simulink model "Nmpc_pathctl_casadi"  (R2022b)
settings: Solver=FixedStepAuto  StartTime=0.0  StopTime=433  FixedStep=.001  MaxStep=0.01  RelTol=1e-3
values from neighbouring files (symbols this model uses):
  xuanze = Input(15)    [NMPC_casadi_yhn.m]    (also in plotfig.m = 0)
libraries: Solver_SF x1
(part 2 of 11)

== matlab function Nmpc_pathctl_casadi/MATLAB Function1 ==
  data: V input; w input; z input; V0 output; lamada input; curvepos0 input; lateralPos0 input; theta0 input; w0 output; lamada0 output; z0 output; Flag output; target input
function [V0,w0, lamada0,z0,Flag]= fcn(V,w,z,lamada,curvepos0,lateralPos0,theta0,target)

V0 = V;
w0 = w;
lamada0 = lamada;
z0 = z;
%% 代入真实的车辆状态，为计算真实的轮胎侧偏角做准备
d = 1.55; %左右轮距
Lf = 1.05;%质心到前轴的距离
Lr = 1.61;%质心到后轴的距离
hcg = 0.54;%质心高度
Iz = 2059.2;%转动惯量
m = 1430;%质量
Iw = 16.8;%车轮转动惯量
Re = 0.3018;%轮胎自由半径
g = 9.8;%重力系数
K_air = 0.9;%空气阻力系数
A = 2.2;%迎风面积
rho_air = 1.206;%空气密度
K_roll = 0.002;%滚动阻力系数
c1f = 1.68;%前轮参数
c1r = 1.49;%后轮参数
c2f = 10.56;%前轮参数
c2r = 15.026;%后轮参数
c3f = 0.02;
c3r = 0.02;
Cy = 1;
Cy_dot = 0.1;
Cs_dot = 0.8;
Cz = 35;
Ctheta_dot = 1;
V_tar = 15;
h = 0.02;
eplim = 50;
epsilon=10^(-6);%epsilon is the tolerance;
min1=5; %min1 & max1 are minimum and maximum number of iterations;
max1=40;
Ep=0.05;%不知道这是什么，为了能跑起来，先设置为和老版一样
kk = 0;
%% 控制器参数
Delt_T =0.02; %[s]
N = 15; %% 15 cuts now delays a bit
Nc = 2;
%% 原有参考轨迹
shape=2.4;%参数名称，用于参考轨迹生成
dx1=25;dx2=21.95;%没有任何实际意义，只是参数名称
dy1=4.05;dy2=5.7;%没有任何实际意义，只是参数名称
Xs1=27.19;Xs2=56.46;%参数名称
N_point = 240;%点的个数
% control_points = [];
X_phi=1:1:N_point;%这个点的区间是根据纵向速度（x_dot）来定的，如果速度为10m/s则区间=10*0.1=1
z1=shape/dx1*(X_phi-Xs1)-shape/2;
z2=shape/dx2*(X_phi-Xs2)-shape/2;
Y_ref=dy1/2.*(1+tanh(z1))-dy2/2.*(1+tanh(z2));
gamma_s = atan2(Y_ref,X_phi);

%% 障碍物信息
    X_obstacle=zeros(1,1);
    X_obstacle(1)=30;

    Y_obstacle=zeros(1,1);
    Y_obstacle(1)=0.5;

%% 计算航向角导数
dot_gamma_s = zeros(N_point);
dot_dot_gamma_s = zeros(N_point);
for i=1:N_point-1
    dot_gamma_s(i) = gamma_s(i+1)-gamma_s(i);
end
    dot_gamma_s(N_point)=dot_gamma_s(N_point-1);
for i=1:N_point-1
    dot_dot_gamma_s(i) = dot_gamma_s(i+1)-dot_gamma_s(i);
end
    dot_dot_gamma_s(N_point)=dot_dot_gamma_s(N_point-1);
%% 寻找距离车辆最近的点
target_dist = sqrt((lateralPos0-Y_ref(target))^2 + (curvepos0-X_phi(target))^2);
for goal = target:target+10
    if goal>length(Y_ref)
        i = goal-length(Y_ref);
    else
        i =goal;
    end
    dist = sqrt((lateralPos0-Y_ref(target))^2 + (curvepos0-X_phi(target))^2);
    if dist < target_dist
        target = i;
        err = target_dist;
        target_dist = dist;
    end
    if dist < 0.07
        target = target+1;
        err = target_dist;
        break;
    end
end
%更新到曲线坐标系中
target0 = target;
curvepos0 = target;
lateralPos0 = target_dist;

%% 使用最优控制方法找到P1,P2,P3
x0 = [0,0,0];
V_dac = [x0(1),x0(2),x0(3);1,0,0;0,1,0;0,0,1];
[mm1,n] = size(V_dac);
Y = ones(n+1,1);
for mm = 1:n+1
    Z = V_dac(mm,1:n);
%==========================================================================下面展开函数myobj_f  ON    
x = Z;
P1 = x(1);
P2 = x(2);
P3 = x(3);
x1 = curvepos0;
x2 = lateralPos0;
x3 = theta0;

for j = 1:N
    fenmu = 1-x2*dot_gamma_s(floor(x1));
    fenzi_a = cos(x3-gamma_s(floor(x1)));
    fenzi_b = sin(x3-gamma_s(floor(x1)));
    %控制量更新
    %求解G(x0)
    H_V_a = 2*Cs_dot*(V0*fenzi_a/fenmu-V_tar)*fenzi_a/fenmu;
    H_V_b = 2*Cy_dot*(V0*fenzi_b^2);
    H_V_c = P1*fenzi_a/fenmu;
    H_V_d = P2*fenzi_b;
    H_V = H_V_a+H_V_b+H_V_c+H_V_d;
    H_w = 2*Ctheta_dot*w0+P3;
    H_z = -Cz/(z0+50)-2*lamada0*z0;
    H_lamada = (x1-30)^2/16+(x2-0.5)^2/4-1-z0^2;
    G_x0 = [H_V;H_w;H_z;H_lamada];
    %求解个G(x0+dotx)
    
    x1_tem = x1+Delt_T*V0*fenzi_a/fenmu;
    x2_tem = x2+Delt_T*V0*fenzi_b;
    x3_tem = x3+Delt_T*w0;
    fenmu_tem = 1-x2_tem*dot_gamma_s(floor(x1_tem));
    fenzi_a_tem = cos(x3_tem-gamma_s(floor(x1_tem)));
    fenzi_b_tem = sin(x3_tem-gamma_s(floor(x1_tem)));
    H_V_a = 2*Cs_dot*(V0*fenzi_a_tem/fenmu_tem-V_tar)*fenzi_a_tem/fenmu_tem;
    H_V_b = 2*Cy_dot*(V0*fenzi_b_tem^2);
    H_V_c = P1*fenzi_a_tem/fenmu_tem;
    H_V_d = P2*fenzi_b_tem;
    H_V_xdot = H_V_a+H_V_b+H_V_c+H_V_d;
    H_w_xdot = 2*Ctheta_dot*w0+P3;
    H_z_xdot = -Cz/(z0+eplim)-2*lamada0*z0;
    H_lamada_dot = (x1_tem-30)^2/16+(x2_tem-0.5)^2/4-1-z0^2;
    G_xdot = [H_V_xdot;H_w_xdot;H_z_xdot;H_lamada_dot];
    G_x_xdot = (G_xdot-G_x0)/0.02;
    %求解G对U的偏导
    G_U_a = 2*Cs_dot*(fenzi_a/fenmu)^2+2*Cy_dot*fenzi_b^2;
    G_U_b = 2*Ctheta_dot;
    G_U_c = -Cz/((z0+eplim)^2)-2*lamada0;
    G_U_d = -2*z0;
    G_U = [G_U_a,0,0,0;0,G_U_b,0,0;0,0,G_U_c,G_U_d;0,0,G_U_d,0];
    %求解u的导数
    dot_u = inv(G_U)*(-G_x_xdot-50*G_x0);
    V0 = V0+dot_u(1)*Delt_T;
    w0 = w0+dot_u(2)*Delt_T;
    z0 = z0+dot_u(3)*Delt_T;
    lamada0 = lamada0+dot_u(4)*Delt_T;
    %开始H对x1求偏导
    H_x1_a = 2*Cs_dot*(V0*fenzi_a/fenmu-V_tar)*(V0*fenzi_b/fenmu*dot_gamma_s(floor(x1))+V0*fenzi_a/fenmu^2*dot_dot_gamma_s(floor(x1)));
    H_x1_b = -2*Cy_dot*(V0^2*fenzi_b*fenzi_a*dot_gamma_s(floor(x1)));
    H_x1_c = P1*V0*fenzi_b/fenzi_a*dot_gamma_s(floor(x1))+V0*fenzi_a/fenmu^2*dot_dot_gamma_s(floor(x1));
    H_x1_d = -P2*V0*fenzi_a*dot_gamma_s(floor(x1));
    H_x1 = H_x1_b+H_x1_a+H_x1_c+H_x1_d;
    %开始H对x2求导
    H_x2_a = 2*Cs_dot*(V0*fenzi_a/fenmu-V_tar)*V0*fenzi_a/fenmu^2*dot_gamma_s(floor(x1));
    H_x2_b = 2*Cy*x2;
    H_x2_c = P1*V0*fenzi_a/fenmu*dot_gamma_s(floor(x1));
    H_x2_d = 2*lamada0*(x2-0.5)/4;
    H_x2 = H_x2_a+H_x2_b+H_x2_c+H_x2_d;
    %开始H对x3求导
    H_x3_a = -2*Cs_dot*(V0*fenzi_a/fenmu-V_tar)*fenzi_a/fenmu;
    H_x3_b = 2*Cy_dot*V0*fenzi_b^2;
    H_x3_c = P1*fenzi_a/fenmu;
    H_x3_d = P2*fenzi_b;
    H_x3 = H_x3_a+H_x3_b+H_x3_c+H_x3_d;
    %更新状态
    x1 = x1+Delt_T*V0*fenzi_a/fenmu;
    x2 = x2+Delt_T*V0*fenzi_b;
    x3 = x3+Delt_T*w0;
end
f = abs(P1)+abs(P2)+abs(P3);
%==========================================================================展开函数myobj_f  OFF
    Y(mm) = f;
end
[mm2,lo] = min(Y);
[mm,hi] = max(Y);
li = hi;
ho = lo;
for mm=1:n+1 %寻找次zuix点
    if mm~=lo && mm~=hi && Y(mm)<=Y(li)
        li=mm;
    end
    if mm~=hi && mm~=lo && Y(mm)>=Y(li)
        ho=mm;
    end
end
cnt=0;
%%开始Nelder-Mead algorithm
while (Y(hi)>Y(lo)+epsilon && cnt<max1) || cnt<min1
    S=zeros(1,n);
    for mm=1:n+1
        S=S+V_dac(mm,1:n);
    end
    M=(S-V_dac(hi,1:n))/n;
    R=2*M-V_dac(hi,1:n);
%==========================================================================下面展开函数myobj_f  ON
x=R;
P1 = x(1);
P2 = x(2);
P3 = x(3);
x1 = curvepos0;
x2 = lateralPos0;
x3 = theta0;
for j = 1:N
    fenmu = 1-x2*dot_gamma_s(floor(x1));
    fenzi_a = cos(x3-gamma_s(floor(x1)));
    fenzi_b = sin(x3-gamma_s(floor(x1)));
    %控制量更新
    %求解G(x0)
    H_V_a = 2*Cs_dot*(V0*fenzi_a/fenmu-V_tar)*fenzi_a/fenmu;
    H_V_b = 2*Cy_dot*(V0*fenzi_b^2);
    H_V_c = P1*fenzi_a/fenmu;
    H_V_d = P2*fenzi_b;
    H_V = H_V_a+H_V_b+H_V_c+H_V_d;
    H_w = 2*Ctheta_dot*w0+P3;
    H_z = -Cz/(z0+50)-2*lamada0*z0;
    H_lamada = (x1-30)^2/16+(x2-0.5)^2/4-1-z0^2;
    G_x0 = [H_V;H_w;H_z;H_lamada];
    %求解个G(x0+dotx)
    x1_tem = x1+Delt_T*V0*fenzi_a/fenmu;
    x2_tem = x2+Delt_T*V0*fenzi_b;
    x3_tem = x3+Delt_T*w0;
    fenmu_tem = 1-x2_tem*dot_gamma_s(floor(x1_tem));
    fenzi_a_tem = cos(x3_tem-gamma_s(floor(x1_tem)));
    fenzi_b_tem = sin(x3_tem-gamma_s(floor(x1_tem)));
    H_V_a = 2*Cs_dot*(V0*fenzi_a_tem/fenmu_tem-V_tar)*fenzi_a_tem/fenmu_tem;
    H_V_b = 2*Cy_dot*(V0*fenzi_b_tem^2);
    H_V_c = P1*fenzi_a_tem/fenmu_tem;
    H_V_d = P2*fenzi_b_tem;
    H_V_xdot = H_V_a+H_V_b+H_V_c+H_V_d;
    H_w_xdot = 2*Ctheta_dot*w0+P3;
    H_z_xdot = -Cz/(z0+eplim)-2*lamada0*z0;
    H_lamada_dot = (x1_tem-30)^2/16+(x2_tem-0.5)^2/4-1-z0^2;
    G_xdot = [H_V_xdot;H_w_xdot;H_z_xdot;H_lamada_dot];
    G_x_xdot = (G_xdot-G_x0)/0.02;
    %求解G对U的偏导
    G_U_a = 2*Cs_dot*(fenzi_a/fenmu)^2+2*Cy_dot*fenzi_b^2;
    G_U_b = 2*Ctheta_dot;
    G_U_c = -Cz/((z0+eplim)^2)-2*lamada0;
    G_U_d = -2*z0;
    G_U = [G_U_a,0,0,0;0,G_U_b,0,0;0,0,G_U_c,G_U_d;0,0,G_U_d,0];
    %求解u的导数
    dot_u = inv(G_U)*(-G_x_xdot-50*G_x0);
    V0 = V0+dot_u(1)*Delt_T;
    w0 = w0+dot_u(2)*Delt_T;
    z0 = z0+dot_u(3)*Delt_T;
    lamada0 = lamada0+dot_u(4)*Delt_T;
    %开始H对x1求偏导
    H_x1_a = 2*Cs_dot*(V0*fenzi_a/fenmu-V_tar)*(V0*fenzi_b/fenmu*dot_gamma_s(floor(x1))+V0*fenzi_a/fenmu^2*dot_dot_gamma_s(floor(x1)));
    H_x1_b = -2*Cy_dot*(V0^2*fenzi_b*fenzi_a*dot_gamma_s(floor(x1)));
    H_x1_c = P1*V0*fenzi_b/fenzi_a*dot_gamma_s(floor(x1))+V0*fenzi_a/fenmu^2*dot_dot_gamma_s(floor(x1));
    H_x1_d = -P2*V0*fenzi_a*dot_gamma_s(floor(x1));
    H_x1 = H_x1_b+H_x1_a+H_x1_c+H_x1_d;
    %开始H对x2求导
    H_x2_a = 2*Cs_dot*(V0*fenzi_a/fenmu-V_tar)*V0*fenzi_a/fenmu^2*dot_gamma_s(floor(x1));
    H_x2_b = 2*Cy*x2;
    H_x2_c = P1*V0*fenzi_a/fenmu*dot_gamma_s(floor(x1));
    H_x2_d = 2*lamada0*(x2-0.5)/4;
    H_x2 = H_x2_a+H_x2_b+H_x2_c+H_x2_d;
    %开始H对x3求导
    H_x3_a = -2*Cs_dot*(V0*fenzi_a/fenmu-V_tar)*fenzi_a/fenmu;
    H_x3_b = 2*Cy_dot*V0*fenzi_b^2;
    H_x3_c = P1*fenzi_a/fenmu;
    H_x3_d = P2*fenzi_b;
    H_x3 = H_x3_a+H_x3_b+H_x3_c+H_x3_d;
    %更新状态
    x1 = x1+Delt_T*V0*fenzi_a/fenmu;
    x2 = x2+Delt_T*V0*fenzi_b;
    x3 = x3+Delt_T*w0;
end
f = abs(P1)+abs(P2)+abs(P3);
%==========================================================================展开函数myobj_f  OFF
yR=f;
    if yR<Y(ho)
        if Y(li)<yR
            V_dac(hi,1:n)=R;
            Y(hi)=yR;
        else
            E=2*R-M;
%==========================================================================下面展开函数myobj_f  ON
x = E;
P1 = x(1);
P2 = x(2);
P3 = x(3);
x1 = curvepos0;
x2 = lateralPos0;
x3 = theta0;
for j = 1:N
    fenmu = 1-x2*dot_gamma_s(floor(x1));
    fenzi_a = cos(x3-gamma_s(floor(x1)));
    fenzi_b = sin(x3-gamma_s(floor(x1)));
    %控制量更新
    %求解G(x0)
    H_V_a = 2*Cs_dot*(V0*fenzi_a/fenmu-V_tar)*fenzi_a/fenmu;
    H_V_b = 2*Cy_dot*(V0*fenzi_b^2);
    H_V_c = P1*fenzi_a/fenmu;
    H_V_d = P2*fenzi_b;
    H_V = H_V_a+H_V_b+H_V_c+H_V_d;
    H_w = 2*Ctheta_dot*w0+P3;
    H_z = -Cz/(z0+50)-2*lamada0*z0;
    H_lamada = (x1-30)^2/16+(x2-0.5)^2/4-1-z0^2;
    G_x0 = [H_V;H_w;H_z;H_lamada];
    %求解个G(x0+dotx)
    x1_tem = x1+Delt_T*V0*fenzi_a/fenmu;
    x2_tem = x2+Delt_T*V0*fenzi_b;
    x3_tem = x3+Delt_T*w0;
    fenmu_tem = 1-x2_tem*dot_gamma_s(floor(x1_tem));
    fenzi_a_tem = cos(x3_tem-gamma_s(floor(x1_tem)));
    fenzi_b_tem = sin(x3_tem-gamma_s(floor(x1_tem)));
    H_V_a = 2*Cs_dot*(V0*fenzi_a_tem/fenmu_tem-V_tar)*fenzi_a_tem/fenmu_tem;
    H_V_b = 2*Cy_dot*(V0*fenzi_b_tem^2);
    H_V_c = P1*fenzi_a_tem/fenmu_tem;
    H_V_d = P2*fenzi_b_tem;
    H_V_xdot = H_V_a+H_V_b+H_V_c+H_V_d;
    H_w_xdot = 2*Ctheta_dot*w0+P3;
    H_z_xdot = -Cz/(z0+eplim)-2*lamada0*z0;
    H_lamada_dot = (x1_tem-30)^2/16+(x2_tem-0.5)^2/4-1-z0^2;
    G_xdot = [H_V_xdot;H_w_xdot;H_z_xdot;H_lamada_dot];
    G_x_xdot = (G_xdot-G_x0)/0.02;
    %求解G对U的偏导
    G_U_a = 2*Cs_dot*(fenzi_a/fenmu)^2+2*Cy_dot*fenzi_b^2;
    G_U_b = 2*Ctheta_dot;
    G_U_c = -Cz/((z0+eplim)^2)-2*lamada0;
    G_U_d = -2*z0;
    G_U = [G_U_a,0,0,0;0,G_U_b,0,0;0,0,G_U_c,G_U_d;0,0,G_U_d,0];
    %求解u的导数
    dot_u = inv(G_U)*(-G_x_xdot-50*G_x0);
    V0 = V0+dot_u(1)*Delt_T;
    w0 = w0+dot_u(2)*Delt_T;
    z0 = z0+dot_u(3)*Delt_T;
    lamada0 = lamada0+dot_u(4)*Delt_T;
    %开始H对x1求偏导
    H_x1_a = 2*Cs_dot*(V0*fenzi_a/fenmu-V_tar)*(V0*fenzi_b/fenmu*dot_gamma_s(floor(x1))+V0*fenzi_a/fenmu^2*dot_dot_gamma_s(floor(x1)));
    H_x1_b = -2*Cy_dot*(V0^2*fenzi_b*fenzi_a*dot_gamma_s(floor(x1)));
    H_x1_c = P1*V0*fenzi_b/fenzi_a*dot_gamma_s(floor(x1))+V0*fenzi_a/fenmu^2*dot_dot_gamma_s(floor(x1));
    H_x1_d = -P2*V0*fenzi_a*dot_gamma_s(floor(x1));
    H_x1 = H_x1_b+H_x1_a+H_x1_c+H_x1_d;
    %开始H对x2求导
    H_x2_a = 2*Cs_dot*(V0*fenzi_a/fenmu-V_tar)*V0*fenzi_a/fenmu^2*dot_gamma_s(floor(x1));
    H_x2_b = 2*Cy*x2;
    H_x2_c = P1*V0*fenzi_a/fenmu*dot_gamma_s(floor(x1));
    H_x2_d = 2*lamada0*(x2-0.5)/4;
    H_x2 = H_x2_a+H_x2_b+H_x2_c+H_x2_d;
    %开始H对x3求导
    H_x3_a = -2*Cs_dot*(V0*fenzi_a/fenmu-V_tar)*fenzi_a/fenmu;
    H_x3_b = 2*Cy_dot*V0*fenzi_b^2;
    H_x3_c = P1*fenzi_a/fenmu;
    H_x3_d = P2*fenzi_b;
    H_x3 = H_x3_a+H_x3_b+H_x3_c+H_x3_d;
    %更新状态
    x1 = x1+Delt_T*V0*fenzi_a/fenmu;
    x2 = x2+Delt_T*V0*fenzi_b;
    x3 = x3+Delt_T*w0;
end
f = abs(P1)+abs(P2)+abs(P3);
%==========================================================================展开函数myobj_f  OFF
            yE=f;
            if yE<Y(li)
                V_dac(hi,1:n)=E;
                Y(hi)=yE;
            else
                V_dac(hi,1:n)=R;
                Y(hi)=yR;
            end
        end
    else
        if yR<Y(hi)
            V_dac(hi,1:n)=R;
            Y(hi)=yR;
        end
        C1_dac=(V_dac(hi,1:n)+M)/2;
%==========================================================================下面展开函数myobj_f  ON
x=C1_dac;
P1 = x(1);
P2 = x(2);
P3 = x(3);
x1 = curvepos0;
x2 = lateralPos0;
x3 = theta0;
for j = 1:N
    fenmu = 1-x2*dot_gamma_s(floor(x1));
    fenzi_a = cos(x3-gamma_s(floor(x1)));
    fenzi_b = sin(x3-gamma_s(floor(x1)));
    %控制量更新
    %求解G(x0)
    H_V_a = 2*Cs_dot*(V0*fenzi_a/fenmu-V_tar)*fenzi_a/fenmu;
    H_V_b = 2*Cy_dot*(V0*fenzi_b^2);
    H_V_c = P1*fenzi_a/fenmu;
    H_V_d = P2*fenzi_b;
    H_V = H_V_a+H_V_b+H_V_c+H_V_d;
    H_w = 2*Ctheta_dot*w0+P3;
    H_z = -Cz/(z0+50)-2*lamada0*z0;
    H_lamada = (x1-30)^2/16+(x2-0.5)^2/4-1-z0^2;
    G_x0 = [H_V;H_w;H_z;H_lamada];
    %求解个G(x0+dotx)
    x1_tem = x1+Delt_T*V0*fenzi_a/fenmu;
    x2_tem = x2+Delt_T*V0*fenzi_b;
    x3_tem = x3+Delt_T*w0;
    fenmu_tem = 1-x2_tem*dot_gamma_s(floor(x1_tem));
    fenzi_a_tem = cos(x3_tem-gamma_s(floor(x1_tem)));
    fenzi_b_tem = sin(x3_tem-gamma_s(floor(x1_tem)));
    H_V_a = 2*Cs_dot*(V0*fenzi_a_tem/fenmu_tem-V_tar)*fenzi_a_tem/fenmu_tem;
    H_V_b = 2*Cy_dot*(V0*fenzi_b_tem^2);
    H_V_c = P1*fenzi_a_tem/fenmu_tem;
    H_V_d = P2*fenzi_b_tem;
    H_V_xdot = H_V_a+H_V_b+H_V_c+H_V_d;
    H_w_xdot = 2*Ctheta_dot*w0+P3;
    H_z_xdot = -Cz/(z0+eplim)-2*lamada0*z0;
    H_lamada_dot = (x1_tem-30)^2/16+(x2_tem-0.5)^2/4-1-z0^2;
    G_xdot = [H_V_xdot;H_w_xdot;H_z_xdot;H_lamada_dot];
    G_x_xdot = (G_xdot-G_x0)/0.02;
    %求解G对U的偏导
    G_U_a = 2*Cs_dot*(fenzi_a/fenmu)^2+2*Cy_dot*fenzi_b^2;
    G_U_b = 2*Ctheta_dot;
    G_U_c = -Cz/((z0+eplim)^2)-2*lamada0;
    G_U_d = -2*z0;
    G_U = [G_U_a,0,0,0;0,G_U_b,0,0;0,0,G_U_c,G_U_d;0,0,G_U_d,0];
    %求解u的导数
    dot_u = inv(G_U)*(-G_x_xdot-50*G_x0);
    V0 = V0+dot_u(1)*Delt_T;
    w0 = w0+dot_u(2)*Delt_T;
    z0 = z0+dot_u(3)*Delt_T;
    lamada0 = lamada0+dot_u(4)*Delt_T;
    %开始H对x1求偏导
    H_x1_a = 2*Cs_dot*(V0*fenzi_a/fenmu-V_tar)*(V0*fenzi_b/fenmu*dot_gamma_s(floor(x1))+V0*fenzi_a/fenmu^2*dot_dot_gamma_s(floor(x1)));
    H_x1_b = -2*Cy_dot*(V0^2*fenzi_b*fenzi_a*dot_gamma_s(floor(x1)));
    H_x1_c = P1*V0*fenzi_b/fenzi_a*dot_gamma_s(floor(x1))+V0*fenzi_a/fenmu^2*dot_dot_gamma_s(floor(x1));
    H_x1_d = -P2*V0*fenzi_a*dot_gamma_s(floor(x1));
    H_x1 = H_x1_b+H_x1_a+H_x1_c+H_x1_d;
    %开始H对x2求导
    H_x2_a = 2*Cs_dot*(V0*fenzi_a/fenmu-V_tar)*V0*fenzi_a/fenmu^2*dot_gamma_s(floor(x1));
    H_x2_b = 2*Cy*x2;
    H_x2_c = P1*V0*fenzi_a/fenmu*dot_gamma_s(floor(x1));
    H_x2_d = 2*lamada0*(x2-0.5)/4;
    H_x2 = H_x2_a+H_x2_b+H_x2_c+H_x2_d;
    %开始H对x3求导
    H_x3_a = -2*Cs_dot*(V0*fenzi_a/fenmu-V_tar)*fenzi_a/fenmu;
    H_x3_b = 2*Cy_dot*V0*fenzi_b^2;
    H_x3_c = P1*fenzi_a/fenmu;
    H_x3_d = P2*fenzi_b;
    H_x3 = H_x3_a+H_x3_b+H_x3_c+H_x3_d;
    %更新状态
    x1 = x1+Delt_T*V0*fenzi_a/fenmu;
    x2 = x2+Delt_T*V0*fenzi_b;
    x3 = x3+Delt_T*w0;
end
f = abs(P1)+abs(P2)+abs(P3);
%==========================================================================展开函数myobj_f  OFF
        yC1=f;
        C2_dac=(M+R)/2;
%==========================================================================下面展开函数myobj_f  ON
x=C2_dac;
P1 = x(1);
P2 = x(2);
P3 = x(3);
x1 = curvepos0;
x2 = lateralPos0;
x3 = theta0;
for j = 1:N
    fenmu = 1-x2*dot_gamma_s(floor(x1));
    fenzi_a = cos(x3-gamma_s(floor(x1)));
    fenzi_b = sin(x3-gamma_s(floor(x1)));
    %控制量更新
    %求解G(x0)
    H_V_a = 2*Cs_dot*(V0*fenzi_a/fenmu-V_tar)*fenzi_a/fenmu;
    H_V_b = 2*Cy_dot*(V0*fenzi_b^2);
    H_V_c = P1*fenzi_a/fenmu;
    H_V_d = P2*fenzi_b;
    H_V = H_V_a+H_V_b+H_V_c+H_V_d;
    H_w = 2*Ctheta_dot*w0+P3;
    H_z = -Cz/(z0+50)-2*lamada0*z0;
    H_lamada = (x1-30)^2/16+(x2-0.5)^2/4-1-z0^2;
    G_x0 = [H_V;H_w;H_z;H_lamada];
    %求解个G(x0+dotx)
    x1_tem = x1+Delt_T*V0*fenzi_a/fenmu;
    x2_tem = x2+Delt_T*V0*fenzi_b;
    x3_tem = x3+Delt_T*w0;
    fenmu_tem = 1-x2_tem*dot_gamma_s(floor(x1_tem));
    fenzi_a_tem = cos(x3_tem-gamma_s(floor(x1_tem)));
    fenzi_b_tem = sin(x3_tem-gamma_s(floor(x1_tem)));
    H_V_a = 2*Cs_dot*(V0*fenzi_a_tem/fenmu_tem-V_tar)*fenzi_a_tem/fenmu_tem;
    H_V_b = 2*Cy_dot*(V0*fenzi_b_tem^2);
    H_V_c = P1*fenzi_a_tem/fenmu_tem;
    H_V_d = P2*fenzi_b_tem;
    H_V_xdot = H_V_a+H_V_b+H_V_c+H_V_d;
    H_w_xdot = 2*Ctheta_dot*w0+P3;
    H_z_xdot = -Cz/(z0+eplim)-2*lamada0*z0;
    H_lamada_dot = (x1_tem-30)^2/16+(x2_tem-0.5)^2/4-1-z0^2;
    G_xdot = [H_V_xdot;H_w_xdot;H_z_xdot;H_lamada_dot];
    G_x_xdot = (G_xdot-G_x0)/0.02;
    %求解G对U的偏导
    G_U_a = 2*Cs_dot*(fenzi_a/fenmu)^2+2*Cy_dot*fenzi_b^2;
    G_U_b = 2*Ctheta_dot;
    G_U_c = -Cz/((z0+eplim)^2)-2*lamada0;
    G_U_d = -2*z0;
    G_U = [G_U_a,0,0,0;0,G_U_b,0,0;0,0,G_U_c,G_U_d;0,0,G_U_d,0];
    %求解u的导数
    dot_u = inv(G_U)*(-G_x_xdot-50*G_x0);
    V0 = V0+dot_u(1)*Delt_T;
    w0 = w0+dot_u(2)*Delt_T;
    z0 = z0+dot_u(3)*Delt_T;
    lamada0 = lamada0+dot_u(4)*Delt_T;
    %开始H对x1求偏导
    H_x1_a = 2*Cs_dot*(V0*fenzi_a/fenmu-V_tar)*(V0*fenzi_b/fenmu*dot_gamma_s(floor(x1))+V0*fenzi_a/fenmu^2*dot_dot_gamma_s(floor(x1)));
    H_x1_b = -2*Cy_dot*(V0^2*fenzi_b*fenzi_a*dot_gamma_s(floor(x1)));
    H_x1_c = P1*V0*fenzi_b/fenzi_a*dot_gamma_s(floor(x1))+V0*fenzi_a/fenmu^2*dot_dot_gamma_s(floor(x1));
    H_x1_d = -P2*V0*fenzi_a*dot_gamma_s(floor(x1));
    H_x1 = H_x1_b+H_x1_a+H_x1_c+H_x1_d;
    %开始H对x2求导
    H_x2_a = 2*Cs_dot*(V0*fenzi_a/fenmu-V_tar)*V0*fenzi_a/fenmu^2*dot_gamma_s(floor(x1));
    H_x2_b = 2*Cy*x2;
    H_x2_c = P1*V0*fenzi_a/fenmu*dot_gamma_s(floor(x1));
    H_x2_d = 2*lamada0*(x2-0.5)/4;
    H_x2 = H_x2_a+H_x2_b+H_x2_c+H_x2_d;
    %开始H对x3求导
    H_x3_a = -2*Cs_dot*(V0*fenzi_a/fenmu-V_tar)*fenzi_a/fenmu;
    H_x3_b = 2*Cy_dot*V0*fenzi_b^2;
    H_x3_c = P1*fenzi_a/fenmu;
    H_x3_d = P2*fenzi_b;
    H_x3 = H_x3_a+H_x3_b+H_x3_c+H_x3_d;
    %更新状态
    x1 = x1+Delt_T*V0*fenzi_a/fenmu;
    x2 = x2+Delt_T*V0*fenzi_b;
    x3 = x3+Delt_T*w0;
end
f = abs(P1)+abs(P2)+abs(P3);
%==========================================================================展开函数myobj_f  OFF
        yC2=f;
        if yC2<yC1
            C1_dac=C2_dac;
            yC1=yC2;
        end
        if yC1<Y(hi)
            V_dac(hi,1:n)=C1_dac;
            Y(hi)=yC1;
        else
            for mm=1:n+1
                if mm~=lo
                    V_dac(mm,1:n)=(V_dac(mm,1:n)+V_dac(lo,1:n))/2;
                    Z=V_dac(mm,1:n);
%==========================================================================下面展开函数myobj_f  ON
x=Z;
P1 = x(1);
P2 = x(2);
P3 = x(3);
x1 = curvepos0;
x2 = lateralPos0;
x3 = theta0;
for j = 1:N
    fenmu = 1-x2*dot_gamma_s(floor(x1));
    fenzi_a = cos(x3-gamma_s(floor(x1)));
    fenzi_b = sin(x3-gamma_s(floor(x1)));
    %控制量更新
    %求解G(x0)
    H_V_a = 2*Cs_dot*(V0*fenzi_a/fenmu-V_tar)*fenzi_a/fenmu;
    H_V_b = 2*Cy_dot*(V0*fenzi_b^2);
    H_V_c = P1*fenzi_a/fenmu;
    H_V_d = P2*fenzi_b;
    H_V = H_V_a+H_V_b+H_V_c+H_V_d;
    H_w = 2*Ctheta_dot*w0+P3;
    H_z = -Cz/(z0+50)-2*lamada0*z0;
    H_lamada = (x1-30)^2/16+(x2-0.5)^2/4-1-z0^2;
    G_x0 = [H_V;H_w;H_z;H_lamada];
    %求解个G(x0+dotx)
    x1_tem = x1+Delt_T*V0*fenzi_a/fenmu;
    x2_tem = x2+Delt_T*V0*fenzi_b;
    x3_tem = x3+Delt_T*w0;
    fenmu_tem = 1-x2_tem*dot_gamma_s(floor(x1_tem));
    fenzi_a_tem = cos(x3_tem-gamma_s(floor(x1_tem)));
    fenzi_b_tem = sin(x3_tem-gamma_s(floor(x1_tem)));
    H_V_a = 2*Cs_dot*(V0*fenzi_a_tem/fenmu_tem-V_tar)*fenzi_a_tem/fenmu_tem;
    H_V_b = 2*Cy_dot*(V0*fenzi_b_tem^2);
    H_V_c = P1*fenzi_a_tem/fenmu_tem;
    H_V_d = P2*fenzi_b_tem;
    H_V_xdot = H_V_a+H_V_b+H_V_c+H_V_d;
    H_w_xdot = 2*Ctheta_dot*w0+P3;
    H_z_xdot = -Cz/(z0+eplim)-2*lamada0*z0;
    H_lamada_dot = (x1_tem-30)^2/16+(x2_tem-0.5)^2/4-1-z0^2;
    G_xdot = [H_V_xdot;H_w_xdot;H_z_xdot;H_lamada_dot];
    G_x_xdot = (G_xdot-G_x0)/0.02;
    %求解G对U的偏导
    G_U_a = 2*Cs_dot*(fenzi_a/fenmu)^2+2*Cy_dot*fenzi_b^2;
    G_U_b = 2*Ctheta_dot;
    G_U_c = -Cz/((z0+eplim)^2)-2*lamada0;
    G_U_d = -2*z0;
    G_U = [G_U_a,0,0,0;0,G_U_b,0,0;0,0,G_U_c,G_U_d;0,0,G_U_d,0];
    %求解u的导数
    dot_u = inv(G_U)*(-G_x_xdot-50*G_x0);
    V0 = V0+dot_u(1)*Delt_T;
    w0 = w0+dot_u(2)*Delt_T;
    z0 = z0+dot_u(3)*Delt_T;
    lamada0 = lamada0+dot_u(4)*Delt_T;
    %开始H对x1求偏导
    H_x1_a = 2*Cs_dot*(V0*fenzi_a/fenmu-V_tar)*(V0*fenzi_b/fenmu*dot_gamma_s(floor(x1))+V0*fenzi_a/fenmu^2*dot_dot_gamma_s(floor(x1)));
    H_x1_b = -2*Cy_dot*(V0^2*fenzi_b*fenzi_a*dot_gamma_s(floor(x1)));
    H_x1_c = P1*V0*fenzi_b/fenzi_a*dot_gamma_s(floor(x1))+V0*fenzi_a/fenmu^2*dot_dot_gamma_s(floor(x1));
    H_x1_d = -P2*V0*fenzi_a*dot_gamma_s(floor(x1));
    H_x1 = H_x1_b+H_x1_a+H_x1_c+H_x1_d;
    %开始H对x2求导
    H_x2_a = 2*Cs_dot*(V0*fenzi_a/fenmu-V_tar)*V0*fenzi_a/fenmu^2*dot_gamma_s(floor(x1));
    H_x2_b = 2*Cy*x2;
    H_x2_c = P1*V0*fenzi_a/fenmu*dot_gamma_s(floor(x1));
    H_x2_d = 2*lamada0*(x2-0.5)/4;
    H_x2 = H_x2_a+H_x2_b+H_x2_c+H_x2_d;
    %开始H对x3求导
    H_x3_a = -2*Cs_dot*(V0*fenzi_a/fenmu-V_tar)*fenzi_a/fenmu;
    H_x3_b = 2*Cy_dot*V0*fenzi_b^2;
    H_x3_c = P1*fenzi_a/fenmu;
    H_x3_d = P2*fenzi_b;
    H_x3 = H_x3_a+H_x3_b+H_x3_c+H_x3_d;
    %更新状态
    x1 = x1+Delt_T*V0*fenzi_a/fenmu;
    x2 = x2+Delt_T*V0*fenzi_b;
    x3 = x3+Delt_T*w0;
end
f = abs(P1)+abs(P2)+abs(P3);
%==========================================================================展开函数myobj_f  OFF
                    Y(mm)=f;
                end
            end
        end
    end
    [mm4,lo]=min(Y);
    [mm5,hi]=max(Y);
    li=hi;
    ho=lo;
    for mm=1:n+1
        if mm~=lo && mm~=hi && Y(mm)<=Y(li)
            li=mm;
        end
        if mm~=hi && mm~=lo && Y(mm)>=Y(li)
            ho=mm;
        end
    end
    cnt=cnt+1;   
end
snorm=0;   
for mm=1:n
    s=norm(V_dac(mm)-V_dac(lo));
    if s>=snorm
        snorm=s; 
    end
end
Re=[V_dac(lo,1:n) cnt];
%==========================================================================下面展开函数myobj_f  ON  
x=[Re(1),Re(2),Re(3)];
P1 = x(1);
P2 = x(2);
P3 = x(3);
x1 = curvepos0;
x2 = lateralPos0;
x3 = theta0;
for j = 1:N
    fenmu = 1-x2*dot_gamma_s(floor(x1));
    fenzi_a = cos(x3-gamma_s(floor(x1)));
    fenzi_b = sin(x3-gamma_s(floor(x1)));
    %控制量更新
    %求解G(x0)
    H_V_a = 2*Cs_dot*(V0*fenzi_a/fenmu-V_tar)*fenzi_a/fenmu;
    H_V_b = 2*Cy_dot*(V0*fenzi_b^2);
    H_V_c = P1*fenzi_a/fenmu;
    H_V_d = P2*fenzi_b;
    H_V = H_V_a+H_V_b+H_V_c+H_V_d;
    H_w = 2*Ctheta_dot*w0+P3;
    H_z = -Cz/(z0+50)-2*lamada0*z0;
    H_lamada = (x1-30)^2/16+(x2-0.5)^2/4-1-z0^2;
    G_x0 = [H_V;H_w;H_z;H_lamada];
    %求解个G(x0+dotx)
    x1_tem = x1+Delt_T*V0*fenzi_a/fenmu;
    x2_tem = x2+Delt_T*V0*fenzi_b;
    x3_tem = x3+Delt_T*w0;
    fenmu_tem = 1-x2_tem*dot_gamma_s(floor(x1_tem));
    fenzi_a_tem = cos(x3_tem-gamma_s(floor(x1_tem)));
    fenzi_b_tem = sin(x3_tem-gamma_s(floor(x1_tem)));
    H_V_a = 2*Cs_dot*(V0*fenzi_a_tem/fenmu_tem-V_tar)*fenzi_a_tem/fenmu_tem;
    H_V_b = 2*Cy_dot*(V0*fenzi_b_tem^2);
    H_V_c = P1*fenzi_a_tem/fenmu_tem;
    H_V_d = P2*fenzi_b_tem;
    H_V_xdot = H_V_a+H_V_b+H_V_c+H_V_d;
    H_w_xdot = 2*Ctheta_dot*w0+P3;
    H_z_xdot = -Cz/(z0+eplim)-2*lamada0*z0;
    H_lamada_dot = (x1_tem-30)^2/16+(x2_tem-0.5)^2/4-1-z0^2;
    G_xdot = [H_V_xdot;H_w_xdot;H_z_xdot;H_lamada_dot];
    G_x_xdot = (G_xdot-G_x0)/0.02;
    %求解G对U的偏导
    G_U_a = 2*Cs_dot*(fenzi_a/fenmu)^2+2*Cy_dot*fenzi_b^2;
    G_U_b = 2*Ctheta_dot;
    G_U_c = -Cz/((z0+eplim)^2)-2*lamada0;
    G_U_d = -2*z0;
    G_U = [G_U_a,0,0,0;0,G_U_b,0,0;0,0,G_U_c,G_U_d;0,0,G_U_d,0];
    %求解u的导数
    dot_u = inv(G_U)*(-G_x_xdot-50*G_x0);
    V0 = V0+dot_u(1)*Delt_T;
    w0 = w0+dot_u(2)*Delt_T;
    z0 = z0+dot_u(3)*Delt_T;
    lamada0 = lamada0+dot_u(4)*Delt_T;
    %开始H对x1求偏导
    H_x1_a = 2*Cs_dot*(V0*fenzi_a/fenmu-V_tar)*(V0*fenzi_b/fenmu*dot_gamma_s(floor(x1))+V0*fenzi_a/fenmu^2*dot_dot_gamma_s(floor(x1)));
    H_x1_b = -2*Cy_dot*(V0^2*fenzi_b*fenzi_a*dot_gamma_s(floor(x1)));
    H_x1_c = P1*V0*fenzi_b/fenzi_a*dot_gamma_s(floor(x1))+V0*fenzi_a/fenmu^2*dot_dot_gamma_s(floor(x1));
    H_x1_d = -P2*V0*fenzi_a*dot_gamma_s(floor(x1));
    H_x1 = H_x1_b+H_x1_a+H_x1_c+H_x1_d;
    %开始H对x2求导
    H_x2_a = 2*Cs_dot*(V0*fenzi_a/fenmu-V_tar)*V0*fenzi_a/fenmu^2*dot_gamma_s(floor(x1));
    H_x2_b = 2*Cy*x2;
    H_x2_c = P1*V0*fenzi_a/fenmu*dot_gamma_s(floor(x1));
    H_x2_d = 2*lamada0*(x2-0.5)/4;
    H_x2 = H_x2_a+H_x2_b+H_x2_c+H_x2_d;
    %开始H对x3求导
    H_x3_a = -2*Cs_dot*(V0*fenzi_a/fenmu-V_tar)*fenzi_a/fenmu;
    H_x3_b = 2*Cy_dot*V0*fenzi_b^2;
    H_x3_c = P1*fenzi_a/fenmu;
    H_x3_d = P2*fenzi_b;
    H_x3 = H_x3_a+H_x3_b+H_x3_c+H_x3_d;
    %更新状态
    x1 = x1+Delt_T*V0*fenzi_a/fenmu;
    x2 = x2+Delt_T*V0*fenzi_b;
    x3 = x3+Delt_T*w0;
end
f = abs(P1)+abs(P2)+abs(P3);
a1 = f;
x_opt1=[Re(1),Re(2),Re(3)];
%==========================================================================展开函数myobj_f  OFF
%% 上面为一个计算循环
if(a1<=Ep)
    x_opt=x_opt1;
    Result_OB=a1;
else %第二个计算循环
    x0=[-1,1,-1];
    V_dac=[x0(1),x0(2),x0(3);1,0,0;0,1,0;0,0,1]; %V_dac is a 3 x n matrix containing starting simplex;
    [mm1 n]=size(V_dac);
% Order the V_dacertices
    Y=ones(n+1,1);
    for mm=1:n+1
        Z=V_dac(mm,1:n);
%==========================================================================下面展开函数myobj_f  ON
x=Z;
P1 = x(1);
P2 = x(2);
P3 = x(3);
x1 = curvepos0;
x2 = lateralPos0;
x3 = theta0;
for j = 1:N
    fenmu = 1-x2*dot_gamma_s(floor(x1));
    fenzi_a = cos(x3-gamma_s(floor(x1)));
    fenzi_b = sin(x3-gamma_s(floor(x1)));
    %控制量更新
    %求解G(x0)
    H_V_a = 2*Cs_dot*(V0*fenzi_a/fenmu-V_tar)*fenzi_a/fenmu;
    H_V_b = 2*Cy_dot*(V0*fenzi_b^2);
    H_V_c = P1*fenzi_a/fenmu;
    H_V_d = P2*fenzi_b;
    H_V = H_V_a+H_V_b+H_V_c+H_V_d;
    H_w = 2*Ctheta_dot*w0+P3;
    H_z = -Cz/(z0+50)-2*lamada0*z0;
    H_lamada = (x1-30)^2/16+(x2-0.5)^2/4-1-z0^2;
    G_x0 = [H_V;H_w;H_z;H_lamada];
    %求解个G(x0+dotx)
    x1_tem = x1+Delt_T*V0*fenzi_a/fenmu;
    x2_tem = x2+Delt_T*V0*fenzi_b;
    x3_tem = x3+Delt_T*w0;
    fenmu_tem = 1-x2_tem*dot_gamma_s(floor(x1_tem));
    fenzi_a_tem = cos(x3_tem-gamma_s(floor(x1_tem)));
    fenzi_b_tem = sin(x3_tem-gamma_s(floor(x1_tem)));
    H_V_a = 2*Cs_dot*(V0*fenzi_a_tem/fenmu_tem-V_tar)*fenzi_a_tem/fenmu_tem;
    H_V_b = 2*Cy_dot*(V0*fenzi_b_tem^2);
    H_V_c = P1*fenzi_a_tem/fenmu_tem;
    H_V_d = P2*fenzi_b_tem;
    H_V_xdot = H_V_a+H_V_b+H_V_c+H_V_d;
    H_w_xdot = 2*Ctheta_dot*w0+P3;
    H_z_xdot = -Cz/(z0+eplim)-2*lamada0*z0;
    H_lamada_dot = (x1_tem-30)^2/16+(x2_tem-0.5)^2/4-1-z0^2;
    G_xdot = [H_V_xdot;H_w_xdot;H_z_xdot;H_lamada_dot];
    G_x_xdot = (G_xdot-G_x0)/0.02;
    %求解G对U的偏导
    G_U_a = 2*Cs_dot*(fenzi_a/fenmu)^2+2*Cy_dot*fenzi_b^2;
    G_U_b = 2*Ctheta_dot;
    G_U_c = -Cz/((z0+eplim)^2)-2*lamada0;
    G_U_d = -2*z0;
    G_U = [G_U_a,0,0,0;0,G_U_b,0,0;0,0,G_U_c,G_U_d;0,0,G_U_d,0];
    %求解u的导数
    dot_u = inv(G_U)*(-G_x_xdot-50*G_x0);
    V0 = V0+dot_u(1)*Delt_T;
    w0 = w0+dot_u(2)*Delt_T;
    z0 = z0+dot_u(3)*Delt_T;
    lamada0 = lamada0+dot_u(4)*Delt_T;
    %开始H对x1求偏导
    H_x1_a = 2*Cs_dot*(V0*fenzi_a/fenmu-V_tar)*(V0*fenzi_b/fenmu*dot_gamma_s(floor(x1))+V0*fenzi_a/fenmu^2*dot_dot_gamma_s(floor(x1)));
    H_x1_b = -2*Cy_dot*(V0^2*fenzi_b*fenzi_a*dot_gamma_s(floor(x1)));
    H_x1_c = P1*V0*fenzi_b/fenzi_a*dot_gamma_s(floor(x1))+V0*fenzi_a/fenmu^2*dot_dot_gamma_s(floor(x1));
    H_x1_d = -P2*V0*fenzi_a*dot_gamma_s(floor(x1));
    H_x1 = H_x1_b+H_x1_a+H_x1_c+H_x1_d;
    %开始H对x2求导
    H_x2_a = 2*Cs_dot*(V0*fenzi_a/fenmu-V_tar)*V0*fenzi_a/fenmu^2*dot_gamma_s(floor(x1));
    H_x2_b = 2*Cy*x2;
    H_x2_c = P1*V0*fenzi_a/fenmu*dot_gamma_s(floor(x1));
    H_x2_d = 2*lamada0*(x2-0.5)/4;
    H_x2 = H_x2_a+H_x2_b+H_x2_c+H_x2_d;
    %开始H对x3求导
    H_x3_a = -2*Cs_dot*(V0*fenzi_a/fenmu-V_tar)*fenzi_a/fenmu;
    H_x3_b = 2*Cy_dot*V0*fenzi_b^2;
    H_x3_c = P1*fenzi_a/fenmu;
    H_x3_d = P2*fenzi_b;
    H_x3 = H_x3_a+H_x3_b+H_x3_c+H_x3_d;
    %更新状态
    x1 = x1+Delt_T*V0*fenzi_a/fenmu;
    x2 = x2+Delt_T*V0*fenzi_b;
    x3 = x3+Delt_T*w0;
end
f = abs(P1)+abs(P2)+abs(P3);
%==========================================================================展开函数myobj_f  OFF
        Y(mm)=f;
    end
    [mm2 lo]=min(Y);
    [mm3 hi]=max(Y);
    li=hi;
    ho=lo;
    for mm=1:n+1
        if mm~=lo && mm~=hi && Y(mm)<=Y(li)
            li=mm;
        end
        if mm~=hi && mm~=lo && Y(mm)>=Y(li)
            ho=mm;
        end
    end
    cnt=0;
%Start of Nelder-Mead algorithm
    while (Y(hi)>Y(lo)+epsilon && cnt<max1) || cnt<min1
        S=zeros(1,n);
        for mm=1:n+1
            S=S+V_dac(mm,1:n);
        end
        M=(S-V_dac(hi,1:n))/n;
        R=2*M-V_dac(hi,1:n);
%==========================================================================下面展开函数myobj_f  ON
x=R;
P1 = x(1);
P2 = x(2);
P3 = x(3);
x1 = curvepos0;
x2 = lateralPos0;
x3 = theta0;
for j = 1:N
    fenmu = 1-x2*dot_gamma_s(floor(x1));
    fenzi_a = cos(x3-gamma_s(floor(x1)));
    fenzi_b = sin(x3-gamma_s(floor(x1)));
    %控制量更新
    %求解G(x0)
    H_V_a = 2*Cs_dot*(V0*fenzi_a/fenmu-V_tar)*fenzi_a/fenmu;
    H_V_b = 2*Cy_dot*(V0*fenzi_b^2);
    H_V_c = P1*fenzi_a/fenmu;
    H_V_d = P2*fenzi_b;
    H_V = H_V_a+H_V_b+H_V_c+H_V_d;
    H_w = 2*Ctheta_dot*w0+P3;
    H_z = -Cz/(z0+50)-2*lamada0*z0;
    H_lamada = (x1-30)^2/16+(x2-0.5)^2/4-1-z0^2;
    G_x0 = [H_V;H_w;H_z;H_lamada];
    %求解个G(x0+dotx)
    x1_tem = x1+Delt_T*V0*fenzi_a/fenmu;
    x2_tem = x2+Delt_T*V0*fenzi_b;
    x3_tem = x3+Delt_T*w0;
    fenmu_tem = 1-x2_tem*dot_gamma_s(floor(x1_tem));
    fenzi_a_tem = cos(x3_tem-gamma_s(floor(x1_tem)));
    fenzi_b_tem = sin(x3_tem-gamma_s(floor(x1_tem)));
    H_V_a = 2*Cs_dot*(V0*fenzi_a_tem/fenmu_tem-V_tar)*fenzi_a_tem/fenmu_tem;
    H_V_b = 2*Cy_dot*(V0*fenzi_b_tem^2);
    H_V_c = P1*fenzi_a_tem/fenmu_tem;
    H_V_d = P2*fenzi_b_tem;
    H_V_xdot = H_V_a+H_V_b+H_V_c+H_V_d;
    H_w_xdot = 2*Ctheta_dot*w0+P3;
    H_z_xdot = -Cz/(z0+eplim)-2*lamada0*z0;
    H_lamada_dot = (x1_tem-30)^2/16+(x2_tem-0.5)^2/4-1-z0^2;
    G_xdot = [H_V_xdot;H_w_xdot;H_z_xdot;H_lamada_dot];
    G_x_xdot = (G_xdot-G_x0)/0.02;
    %求解G对U的偏导
    G_U_a = 2*Cs_dot*(fenzi_a/fenmu)^2+2*Cy_dot*fenzi_b^2;
    G_U_b = 2*Ctheta_dot;
    G_U_c = -Cz/((z0+eplim)^2)-2*lamada0;
    G_U_d = -2*z0;
    G_U = [G_U_a,0,0,0;0,G_U_b,0,0;0,0,G_U_c,G_U_d;0,0,G_U_d,0];
    %求解u的导数
    dot_u = inv(G_U)*(-G_x_xdot-50*G_x0);
    V0 = V0+dot_u(1)*Delt_T;
    w0 = w0+dot_u(2)*Delt_T;
    z0 = z0+dot_u(3)*Delt_T;
    lamada0 = lamada0+dot_u(4)*Delt_T;
    %开始H对x1求偏导
    H_x1_a = 2*Cs_dot*(V0*fenzi_a/fenmu-V_tar)*(V0*fenzi_b/fenmu*dot_gamma_s(floor(x1))+V0*fenzi_a/fenmu^2*dot_dot_gamma_s(floor(x1)));
    H_x1_b = -2*Cy_dot*(V0^2*fenzi_b*fenzi_a*dot_gamma_s(floor(x1)));
    H_x1_c = P1*V0*fenzi_b/fenzi_a*dot_gamma_s(floor(x1))+V0*fenzi_a/fenmu^2*dot_dot_gamma_s(floor(x1));
    H_x1_d = -P2*V0*fenzi_a*dot_gamma_s(floor(x1));
    H_x1 = H_x1_b+H_x1_a+H_x1_c+H_x1_d;
    %开始H对x2求导
    H_x2_a = 2*Cs_dot*(V0*fenzi_a/fenmu-V_tar)*V0*fenzi_a/fenmu^2*dot_gamma_s(floor(x1));
    H_x2_b = 2*Cy*x2;
    H_x2_c = P1*V0*fenzi_a/fenmu*dot_gamma_s(floor(x1));
    H_x2_d = 2*lamada0*(x2-0.5)/4;
    H_x2 = H_x2_a+H_x2_b+H_x2_c+H_x2_d;
    %开始H对x3求导
    H_x3_a = -2*Cs_dot*(V0*fenzi_a/fenmu-V_tar)*fenzi_a/fenmu;
    H_x3_b = 2*Cy_dot*V0*fenzi_b^2;
    H_x3_c = P1*fenzi_a/fenmu;
    H_x3_d = P2*fenzi_b;
    H_x3 = H_x3_a+H_x3_b+H_x3_c+H_x3_d;
    %更新状态
    x1 = x1+Delt_T*V0*fenzi_a/fenmu;
    x2 = x2+Delt_T*V0*fenzi_b;
    x3 = x3+Delt_T*w0;
end
f = abs(P1)+abs(P2)+abs(P3);
%==========================================================================展开函数myobj_f  OFF
        yR=f;
        if yR<Y(ho)
            if Y(li)<yR
                V_dac(hi,1:n)=R;
                Y(hi)=yR;
            else
                E=2*R-M;
%==========================================================================下面展开函数myobj_f  ON
x=E;
P1 = x(1);
P2 = x(2);
P3 = x(3);
x1 = curvepos0;
x2 = lateralPos0;
x3 = theta0;
for j = 1:N
    fenmu = 1-x2*dot_gamma_s(floor(x1));
    fenzi_a = cos(x3-gamma_s(floor(x1)));
    fenzi_b = sin(x3-gamma_s(floor(x1)));
    %控制量更新
    %求解G(x0)
    H_V_a = 2*Cs_dot*(V0*fenzi_a/fenmu-V_tar)*fenzi_a/fenmu;
    H_V_b = 2*Cy_dot*(V0*fenzi_b^2);
    H_V_c = P1*fenzi_a/fenmu;
    H_V_d = P2*fenzi_b;
    H_V = H_V_a+H_V_b+H_V_c+H_V_d;
    H_w = 2*Ctheta_dot*w0+P3;
    H_z = -Cz/(z0+50)-2*lamada0*z0;
    H_lamada = (x1-30)^2/16+(x2-0.5)^2/4-1-z0^2;
    G_x0 = [H_V;H_w;H_z;H_lamada];
    %求解个G(x0+dotx)
    x1_tem = x1+Delt_T*V0*fenzi_a/fenmu;
    x2_tem = x2+Delt_T*V0*fenzi_b;
    x3_tem = x3+Delt_T*w0;
    fenmu_tem = 1-x2_tem*dot_gamma_s(floor(x1_tem));
    fenzi_a_tem = cos(x3_tem-gamma_s(floor(x1_tem)));
    fenzi_b_tem = sin(x3_tem-gamma_s(floor(x1_tem)));
    H_V_a = 2*Cs_dot*(V0*fenzi_a_tem/fenmu_tem-V_tar)*fenzi_a_tem/fenmu_tem;
    H_V_b = 2*Cy_dot*(V0*fenzi_b_tem^2);
    H_V_c = P1*fenzi_a_tem/fenmu_tem;
    H_V_d = P2*fenzi_b_tem;
    H_V_xdot = H_V_a+H_V_b+H_V_c+H_V_d;
    H_w_xdot = 2*Ctheta_dot*w0+P3;
    H_z_xdot = -Cz/(z0+eplim)-2*lamada0*z0;
    H_lamada_dot = (x1_tem-30)^2/16+(x2_tem-0.5)^2/4-1-z0^2;
    G_xdot = [H_V_xdot;H_w_xdot;H_z_xdot;H_lamada_dot];
    G_x_xdot = (G_xdot-G_x0)/0.02;
    %求解G对U的偏导
    G_U_a = 2*Cs_dot*(fenzi_a/fenmu)^2+2*Cy_dot*fenzi_b^2;
    G_U_b = 2*Ctheta_dot;
    G_U_c = -Cz/((z0+eplim)^2)-2*lamada0;
    G_U_d = -2*z0;
    G_U = [G_U_a,0,0,0;0,G_U_b,0,0;0,0,G_U_c,G_U_d;0,0,G_U_d,0];
    %求解u的导数
    dot_u = inv(G_U)*(-G_x_xdot-50*G_x0);
    V0 = V0+dot_u(1)*Delt_T;
    w0 = w0+dot_u(2)*Delt_T;
    z0 = z0+dot_u(3)*Delt_T;
    lamada0 = lamada0+dot_u(4)*Delt_T;
    %开始H对x1求偏导
    H_x1_a = 2*Cs_dot*(V0*fenzi_a/fenmu-V_tar)*(V0*fenzi_b/fenmu*dot_gamma_s(floor(x1))+V0*fenzi_a/fenmu^2*dot_dot_gamma_s(floor(x1)));
    H_x1_b = -2*Cy_dot*(V0^2*fenzi_b*fenzi_a*dot_gamma_s(floor(x1)));
    H_x1_c = P1*V0*fenzi_b/fenzi_a*dot_gamma_s(floor(x1))+V0*fenzi_a/fenmu^2*dot_dot_gamma_s(floor(x1));
    H_x1_d = -P2*V0*fenzi_a*dot_gamma_s(floor(x1));
    H_x1 = H_x1_b+H_x1_a+H_x1_c+H_x1_d;
    %开始H对x2求导
    H_x2_a = 2*Cs_dot*(V0*fenzi_a/fenmu-V_tar)*V0*fenzi_a/fenmu^2*dot_gamma_s(floor(x1));
    H_x2_b = 2*Cy*x2;
    H_x2_c = P1*V0*fenzi_a/fenmu*dot_gamma_s(floor(x1));
    H_x2_d = 2*lamada0*(x2-0.5)/4;
    H_x2 = H_x2_a+H_x2_b+H_x2_c+H_x2_d;
    %开始H对x3求导
    H_x3_a = -2*Cs_dot*(V0*fenzi_a/fenmu-V_tar)*fenzi_a/fenmu;
    H_x3_b = 2*Cy_dot*V0*fenzi_b^2;
    H_x3_c = P1*fenzi_a/fenmu;
    H_x3_d = P2*fenzi_b;
    H_x3 = H_x3_a+H_x3_b+H_x3_c+H_x3_d;
    %更新状态
    x1 = x1+Delt_T*V0*fenzi_a/fenmu;
    x2 = x2+Delt_T*V0*fenzi_b;
    x3 = x3+Delt_T*w0;
end
f = abs(P1)+abs(P2)+abs(P3);
%==========================================================================展开函数myobj_f  OFF
                yE=f;
                if yE<Y(li)
                    V_dac(hi,1:n)=E;
                    Y(hi)=yE;
                else
                    V_dac(hi,1:n)=R;
                    Y(hi)=yR;
                end
            end
        else
            if yR<Y(hi)
                V_dac(hi,1:n)=R;
                Y(hi)=yR;
            end
            C1_dac=(V_dac(hi,1:n)+M)/2;
%==========================================================================下面展开函数myobj_f  ON
x=C1_dac;
P1 = x(1);
P2 = x(2);
P3 = x(3);
x1 = curvepos0;
x2 = lateralPos0;
x3 = theta0;
for j = 1:N
    fenmu = 1-x2*dot_gamma_s(floor(x1));
    fenzi_a = cos(x3-gamma_s(floor(x1)));
    fenzi_b = sin(x3-gamma_s(floor(x1)));
    %控制量更新
    %求解G(x0)
    H_V_a = 2*Cs_dot*(V0*fenzi_a/fenmu-V_tar)*fenzi_a/fenmu;
    H_V_b = 2*Cy_dot*(V0*fenzi_b^2);
    H_V_c = P1*fenzi_a/fenmu;
    H_V_d = P2*fenzi_b;
    H_V = H_V_a+H_V_b+H_V_c+H_V_d;
    H_w = 2*Ctheta_dot*w0+P3;
    H_z = -Cz/(z0+50)-2*lamada0*z0;
    H_lamada = (x1-30)^2/16+(x2-0.5)^2/4-1-z0^2;
    G_x0 = [H_V;H_w;H_z;H_lamada];
    %求解个G(x0+dotx)
    x1_tem = x1+Delt_T*V0*fenzi_a/fenmu;
    x2_tem = x2+Delt_T*V0*fenzi_b;
    x3_tem = x3+Delt_T*w0;
    fenmu_tem = 1-x2_tem*dot_gamma_s(floor(x1_tem));
    fenzi_a_tem = cos(x3_tem-gamma_s(floor(x1_tem)));
    fenzi_b_tem = sin(x3_tem-gamma_s(floor(x1_tem)));
    H_V_a = 2*Cs_dot*(V0*fenzi_a_tem/fenmu_tem-V_tar)*fenzi_a_tem/fenmu_tem;
    H_V_b = 2*Cy_dot*(V0*fenzi_b_tem^2);
    H_V_c = P1*fenzi_a_tem/fenmu_tem;
    H_V_d = P2*fenzi_b_tem;
    H_V_xdot = H_V_a+H_V_b+H_V_c+H_V_d;
    H_w_xdot = 2*Ctheta_dot*w0+P3;
    H_z_xdot = -Cz/(z0+eplim)-2*lamada0*z0;
    H_lamada_dot = (x1_tem-30)^2/16+(x2_tem-0.5)^2/4-1-z0^2;
    G_xdot = [H_V_xdot;H_w_xdot;H_z_xdot;H_lamada_dot];
    G_x_xdot = (G_xdot-G_x0)/0.02;
    %求解G对U的偏导
    G_U_a = 2*Cs_dot*(fenzi_a/fenmu)^2+2*Cy_dot*fenzi_b^2;
    G_U_b = 2*Ctheta_dot;
    G_U_c = -Cz/((z0+eplim)^2)-2*lamada0;
    G_U_d = -2*z0;
    G_U = [G_U_a,0,0,0;0,G_U_b,0,0;0,0,G_U_c,G_U_d;0,0,G_U_d,0];
    %求解u的导数
    dot_u = inv(G_U)*(-G_x_xdot-50*G_x0);
    V0 = V0+dot_u(1)*Delt_T;
    w0 = w0+dot_u(2)*Delt_T;
    z0 = z0+dot_u(3)*Delt_T;
    lamada0 = lamada0+dot_u(4)*Delt_T;
    %开始H对x1求偏导
    H_x1_a = 2*Cs_dot*(V0*fenzi_a/fenmu-V_tar)*(V0*fenzi_b/fenmu*dot_gamma_s(floor(x1))+V0*fenzi_a/fenmu^2*dot_dot_gamma_s(floor(x1)));
    H_x1_b = -2*Cy_dot*(V0^2*fenzi_b*fenzi_a*dot_gamma_s(floor(x1)));
    H_x1_c = P1*V0*fenzi_b/fenzi_a*dot_gamma_s(floor(x1))+V0*fenzi_a/fenmu^2*dot_dot_gamma_s(floor(x1));
    H_x1_d = -P2*V0*fenzi_a*dot_gamma_s(floor(x1));
    H_x1 = H_x1_b+H_x1_a+H_x1_c+H_x1_d;
    %开始H对x2求导
    H_x2_a = 2*Cs_dot*(V0*fenzi_a/fenmu-V_tar)*V0*fenzi_a/fenmu^2*dot_gamma_s(floor(x1));
    H_x2_b = 2*Cy*x2;
    H_x2_c = P1*V0*fenzi_a/fenmu*dot_gamma_s(floor(x1));
    H_x2_d = 2*lamada0*(x2-0.5)/4;
    H_x2 = H_x2_a+H_x2_b+H_x2_c+H_x2_d;
    %开始H对x3求导
    H_x3_a = -2*Cs_dot*(V0*fenzi_a/fenmu-V_tar)*fenzi_a/fenmu;
    H_x3_b = 2*Cy_dot*V0*fenzi_b^2;
    H_x3_c = P1*fenzi_a/fenmu;
    H_x3_d = P2*fenzi_b;
    H_x3 = H_x3_a+H_x3_b+H_x3_c+H_x3_d;
    %更新状态
    x1 = x1+Delt_T*V0*fenzi_a/fenmu;
    x2 = x2+Delt_T*V0*fenzi_b;
    x3 = x3+Delt_T*w0;
end
f = abs(P1)+abs(P2)+abs(P3);
%==========================================================================展开函数myobj_f  OFF
            yC1=f;
            C2_dac=(M+R)/2;
%==========================================================================下面展开函数myobj_f  ON
x=C2_dac;
P1 = x(1);
P2 = x(2);
P3 = x(3);
x1 = curvepos0;
x2 = lateralPos0;
x3 = theta0;
for j = 1:N
    fenmu = 1-x2*dot_gamma_s(floor(x1));
    fenzi_a = cos(x3-gamma_s(floor(x1)));
    fenzi_b = sin(x3-gamma_s(floor(x1)));
    %控制量更新
    %求解G(x0)
    H_V_a = 2*Cs_dot*(V0*fenzi_a/fenmu-V_tar)*fenzi_a/fenmu;
    H_V_b = 2*Cy_dot*(V0*fenzi_b^2);
    H_V_c = P1*fenzi_a/fenmu;
    H_V_d = P2*fenzi_b;
    H_V = H_V_a+H_V_b+H_V_c+H_V_d;
    H_w = 2*Ctheta_dot*w0+P3;
    H_z = -Cz/(z0+50)-2*lamada0*z0;
    H_lamada = (x1-30)^2/16+(x2-0.5)^2/4-1-z0^2;
    G_x0 = [H_V;H_w;H_z;H_lamada];
    %求解个G(x0+dotx)
    x1_tem = x1+Delt_T*V0*fenzi_a/fenmu;
    x2_tem = x2+Delt_T*V0*fenzi_b;
    x3_tem = x3+Delt_T*w0;
    fenmu_tem = 1-x2_tem*dot_gamma_s(floor(x1_tem));
    fenzi_a_tem = cos(x3_tem-gamma_s(floor(x1_tem)));
    fenzi_b_tem = sin(x3_tem-gamma_s(floor(x1_tem)));
    H_V_a = 2*Cs_dot*(V0*fenzi_a_tem/fenmu_tem-V_tar)*fenzi_a_tem/fenmu_tem;
    H_V_b = 2*Cy_dot*(V0*fenzi_b_tem^2);
    H_V_c = P1*fenzi_a_tem/fenmu_tem;
    H_V_d = P2*fenzi_b_tem;
    H_V_xdot = H_V_a+H_V_b+H_V_c+H_V_d;
    H_w_xdot = 2*Ctheta_dot*w0+P3;
    H_z_xdot = -Cz/(z0+eplim)-2*lamada0*z0;
    H_lamada_dot = (x1_tem-30)^2/16+(x2_tem-0.5)^2/4-1-z0^2;
    G_xdot = [H_V_xdot;H_w_xdot;H_z_xdot;H_lamada_dot];
    G_x_xdot = (G_xdot-G_x0)/0.02;
    %求解G对U的偏导
    G_U_a = 2*Cs_dot*(fenzi_a/fenmu)^2+2*Cy_dot*fenzi_b^2;
    G_U_b = 2*Ctheta_dot;
    G_U_c = -Cz/((z0+eplim)^2)-2*lamada0;
    G_U_d = -2*z0;
    G_U = [G_U_a,0,0,0;0,G_U_b,0,0;0,0,G_U_c,G_U_d;0,0,G_U_d,0];
    %求解u的导数
    dot_u = inv(G_U)*(-G_x_xdot-50*G_x0);
    V0 = V0+dot_u(1)*Delt_T;
    w0 = w0+dot_u(2)*Delt_T;
    z0 = z0+dot_u(3)*Delt_T;
    lamada0 = lamada0+dot_u(4)*Delt_T;
    %开始H对x1求偏导
    H_x1_a = 2*Cs_dot*(V0*fenzi_a/fenmu-V_tar)*(V0*fenzi_b/fenmu*dot_gamma_s(floor(x1))+V0*fenzi_a/fenmu^2*dot_dot_gamma_s(floor(x1)));
    H_x1_b = -2*Cy_dot*(V0^2*fenzi_b*fenzi_a*dot_gamma_s(floor(x1)));
    H_x1_c = P1*V0*fenzi_b/fenzi_a*dot_gamma_s(floor(x1))+V0*fenzi_a/fenmu^2*dot_dot_gamma_s(floor(x1));
    H_x1_d = -P2*V0*fenzi_a*dot_gamma_s(floor(x1));
    H_x1 = H_x1_b+H_x1_a+H_x1_c+H_x1_d;
    %开始H对x2求导
    H_x2_a = 2*Cs_dot*(V0*fenzi_a/fenmu-V_tar)*V0*fenzi_a/fenmu^2*dot_gamma_s(floor(x1));
    H_x2_b = 2*Cy*x2;
    H_x2_c = P1*V0*fenzi_a/fenmu*dot_gamma_s(floor(x1));
    H_x2_d = 2*lamada0*(x2-0.5)/4;
    H_x2 = H_x2_a+H_x2_b+H_x2_c+H_x2_d;
    %开始H对x3求导
    H_x3_a = -2*Cs_dot*(V0*fenzi_a/fenmu-V_tar)*fenzi_a/fenmu;
    H_x3_b = 2*Cy_dot*V0*fenzi_b^2;
    H_x3_c = P1*fenzi_a/fenmu;
    H_x3_d = P2*fenzi_b;
    H_x3 = H_x3_a+H_x3_b+H_x3_c+H_x3_d;
    %更新状态
    x1 = x1+Delt_T*V0*fenzi_a/fenmu;
    x2 = x2+Delt_T*V0*fenzi_b;
    x3 = x3+Delt_T*w0;
end
f = abs(P1)+abs(P2)+abs(P3);
%==========================================================================展开函数myobj_f  OFF
            yC2=f;
            if yC2<yC1
                C1_dac=C2_dac;
                yC1=yC2;
            end
            if yC1<Y(hi)
                V_dac(hi,1:n)=C1_dac;
                Y(hi)=yC1;
            else
                for mm=1:n+1
                    if mm~=lo
                        V_dac(mm,1:n)=(V_dac(mm,1:n)+V_dac(lo,1:n))/2;
                        Z=V_dac(mm,1:n);
%==========================================================================下面展开函数myobj_f  ON
x=Z;
P1 = x(1);
P2 = x(2);
P3 = x(3);
x1 = curvepos0;
x2 = lateralPos0;
x3 = theta0;
for j = 1:N
    fenmu = 1-x2*dot_gamma_s(floor(x1));
    fenzi_a = cos(x3-gamma_s(floor(x1)));
    fenzi_b = sin(x3-gamma_s(floor(x1)));
    %控制量更新
    %求解G(x0)
    H_V_a = 2*Cs_dot*(V0*fenzi_a/fenmu-V_tar)*fenzi_a/fenmu;
    H_V_b = 2*Cy_dot*(V0*fenzi_b^2);
    H_V_c = P1*fenzi_a/fenmu;
    H_V_d = P2*fenzi_b;
    H_V = H_V_a+H_V_b+H_V_c+H_V_d;
    H_w = 2*Ctheta_dot*w0+P3;
    H_z = -Cz/(z0+50)-2*lamada0*z0;
    H_lamada = (x1-30)^2/16+(x2-0.5)^2/4-1-z0^2;
    G_x0 = [H_V;H_w;H_z;H_lamada];
    %求解个G(x0+dotx)
    x1_tem = x1+Delt_T*V0*fenzi_a/fenmu;
    x2_tem = x2+Delt_T*V0*fenzi_b;
    x3_tem = x3+Delt_T*w0;
    fenmu_tem = 1-x2_tem*dot_gamma_s(floor(x1_tem));
    fenzi_a_tem = cos(x3_tem-gamma_s(floor(x1_tem)));
    fenzi_b_tem = sin(x3_tem-gamma_s(floor(x1_tem)));
    H_V_a = 2*Cs_dot*(V0*fenzi_a_tem/fenmu_tem-V_tar)*fenzi_a_tem/fenmu_tem;
    H_V_b = 2*Cy_dot*(V0*fenzi_b_tem^2);
    H_V_c = P1*fenzi_a_tem/fenmu_tem;
    H_V_d = P2*fenzi_b_tem;
    H_V_xdot = H_V_a+H_V_b+H_V_c+H_V_d;
    H_w_xdot = 2*Ctheta_dot*w0+P3;
    H_z_xdot = -Cz/(z0+eplim)-2*lamada0*z0;
    H_lamada_dot = (x1_tem-30)^2/16+(x2_tem-0.5)^2/4-1-z0^2;
    G_xdot = [H_V_xdot;H_w_xdot;H_z_xdot;H_lamada_dot];
    G_x_xdot = (G_xdot-G_x0)/0.02;
    %求解G对U的偏导
    G_U_a = 2*Cs_dot*(fenzi_a/fenmu)^2+2*Cy_dot*fenzi_b^2;
    G_U_b = 2*Ctheta_dot;
    G_U_c = -Cz/((z0+eplim)^2)-2*lamada0;
    G_U_d = -2*z0;
    G_U = [G_U_a,0,0,0;0,G_U_b,0,0;0,0,G_U_c,G_U_d;0,0,G_U_d,0];
    %求解u的导数
    dot_u = inv(G_U)*(-G_x_xdot-50*G_x0);
    V0 = V0+dot_u(1)*Delt_T;
    w0 = w0+dot_u(2)*Delt_T;
    z0 = z0+dot_u(3)*Delt_T;
    lamada0 = lamada0+dot_u(4)*Delt_T;
    %开始H对x1求偏导
    H_x1_a = 2*Cs_dot*(V0*fenzi_a/fenmu-V_tar)*(V0*fenzi_b/fenmu*dot_gamma_s(floor(x1))+V0*fenzi_a/fenmu^2*dot_dot_gamma_s(floor(x1)));
    H_x1_b = -2*Cy_dot*(V0^2*fenzi_b*fenzi_a*dot_gamma_s(floor(x1)));
    H_x1_c = P1*V0*fenzi_b/fenzi_a*dot_gamma_s(floor(x1))+V0*fenzi_a/fenmu^2*dot_dot_gamma_s(floor(x1));
    H_x1_d = -P2*V0*fenzi_a*dot_gamma_s(floor(x1));
    H_x1 = H_x1_b+H_x1_a+H_x1_c+H_x1_d;
    %开始H对x2求导
    H_x2_a = 2*Cs_dot*(V0*fenzi_a/fenmu-V_tar)*V0*fenzi_a/fenmu^2*dot_gamma_s(floor(x1));
    H_x2_b = 2*Cy*x2;
    H_x2_c = P1*V0*fenzi_a/fenmu*dot_gamma_s(floor(x1));
    H_x2_d = 2*lamada0*(x2-0.5)/4;
    H_x2 = H_x2_a+H_x2_b+H_x2_c+H_x2_d;
    %开始H对x3求导
    H_x3_a = -2*Cs_dot*(V0*fenzi_a/fenmu-V_tar)*fenzi_a/fenmu;
    H_x3_b = 2*Cy_dot*V0*fenzi_b^2;
    H_x3_c = P1*fenzi_a/fenmu;
    H_x3_d = P2*fenzi_b;
    H_x3 = H_x3_a+H_x3_b+H_x3_c+H_x3_d;
    %更新状态
    x1 = x1+Delt_T*V0*fenzi_a/fenmu;
    x2 = x2+Delt_T*V0*fenzi_b;
    x3 = x3+Delt_T*w0;
end
f = abs(P1)+abs(P2)+abs(P3);
%==========================================================================展开函数myobj_f  OFF
                        Y(mm)=f;
                    end
                end
            end
        end
        [mm4,lo]=min(Y);
        [mm5,hi]=max(Y);
        li=hi;
        ho=lo;
        for mm=1:n+1
            if mm~=lo && mm~=hi && Y(mm)<=Y(li)
                li=mm;
            end
            if mm~=hi && mm~=lo && Y(mm)>=Y(li)
                ho=mm;
            end
        end
        cnt=cnt+1;
    end
    snorm=0;
    for mm=1:n+1
        s=norm(V_dac(mm)-V_dac(lo));
        if s>=snorm
            snorm=s;
        end
    end
    Re=[V_dac(lo,1:n) cnt];
%==========================================================================下面展开函数myobj_f  ON
x=[Re(1),Re(2),Re(3)];
P1 = x(1);
P2 = x(2);
P3 = x(3);
x1 = curvepos0;
x2 = lateralPos0;
x3 = theta0;
for j = 1:N
    fenmu = 1-x2*dot_gamma_s(floor(x1));
    fenzi_a = cos(x3-gamma_s(floor(x1)));
    fenzi_b = sin(x3-gamma_s(floor(x1)));
    %控制量更新
    %求解G(x0)
    H_V_a = 2*Cs_dot*(V0*fenzi_a/fenmu-V_tar)*fenzi_a/fenmu;
    H_V_b = 2*Cy_dot*(V0*fenzi_b^2);
    H_V_c = P1*fenzi_a/fenmu;
    H_V_d = P2*fenzi_b;
    H_V = H_V_a+H_V_b+H_V_c+H_V_d;
    H_w = 2*Ctheta_dot*w0+P3;
    H_z = -Cz/(z0+50)-2*lamada0*z0;
    H_lamada = (x1-30)^2/16+(x2-0.5)^2/4-1-z0^2;
    G_x0 = [H_V;H_w;H_z;H_lamada];
    %求解个G(x0+dotx)
    x1_tem = x1+Delt_T*V0*fenzi_a/fenmu;
    x2_tem = x2+Delt_T*V0*fenzi_b;
    x3_tem = x3+Delt_T*w0;
    fenmu_tem = 1-x2_tem*dot_gamma_s(floor(x1_tem));
    fenzi_a_tem = cos(x3_tem-gamma_s(floor(x1_tem)));
    fenzi_b_tem = sin(x3_tem-gamma_s(floor(x1_tem)));
    H_V_a = 2*Cs_dot*(V0*fenzi_a_tem/fenmu_tem-V_tar)*fenzi_a_tem/fenmu_tem;
    H_V_b = 2*Cy_dot*(V0*fenzi_b_tem^2);
    H_V_c = P1*fenzi_a_tem/fenmu_tem;
    H_V_d = P2*fenzi_b_tem;
    H_V_xdot = H_V_a+H_V_b+H_V_c+H_V_d;
    H_w_xdot = 2*Ctheta_dot*w0+P3;
    H_z_xdot = -Cz/(z0+eplim)-2*lamada0*z0;
    H_lamada_dot = (x1_tem-30)^2/16+(x2_tem-0.5)^2/4-1-z0^2;
    G_xdot = [H_V_xdot;H_w_xdot;H_z_xdot;H_lamada_dot];
    G_x_xdot = (G_xdot-G_x0)/0.02;
    %求解G对U的偏导
    G_U_a = 2*Cs_dot*(fenzi_a/fenmu)^2+2*Cy_dot*fenzi_b^2;
    G_U_b = 2*Ctheta_dot;
    G_U_c = -Cz/((z0+eplim)^2)-2*lamada0;
    G_U_d = -2*z0;
    G_U = [G_U_a,0,0,0;0,G_U_b,0,0;0,0,G_U_c,G_U_d;0,0,G_U_d,0];
    %求解u的导数
    dot_u = inv(G_U)*(-G_x_xdot-50*G_x0);
    V0 = V0+dot_u(1)*Delt_T;
    w0 = w0+dot_u(2)*Delt_T;
    z0 = z0+dot_u(3)*Delt_T;
    lamada0 = lamada0+dot_u(4)*Delt_T;
    %开始H对x1求偏导
    H_x1_a = 2*Cs_dot*(V0*fenzi_a/fenmu-V_tar)*(V0*fenzi_b/fenmu*dot_gamma_s(floor(x1))+V0*fenzi_a/fenmu^2*dot_dot_gamma_s(floor(x1)));
    H_x1_b = -2*Cy_dot*(V0^2*fenzi_b*fenzi_a*dot_gamma_s(floor(x1)));
    H_x1_c = P1*V0*fenzi_b/fenzi_a*dot_gamma_s(floor(x1))+V0*fenzi_a/fenmu^2*dot_dot_gamma_s(floor(x1));
    H_x1_d = -P2*V0*fenzi_a*dot_gamma_s(floor(x1));
    H_x1 = H_x1_b+H_x1_a+H_x1_c+H_x1_d;
    %开始H对x2求导
    H_x2_a = 2*Cs_dot*(V0*fenzi_a/fenmu-V_tar)*V0*fenzi_a/fenmu^2*dot_gamma_s(floor(x1));
    H_x2_b = 2*Cy*x2;
    H_x2_c = P1*V0*fenzi_a/fenmu*dot_gamma_s(floor(x1));
    H_x2_d = 2*lamada0*(x2-0.5)/4;
    H_x2 = H_x2_a+H_x2_b+H_x2_c+H_x2_d;
    %开始H对x3求导
    H_x3_a = -2*Cs_dot*(V0*fenzi_a/fenmu-V_tar)*fenzi_a/fenmu;
    H_x3_b = 2*Cy_dot*V0*fenzi_b^2;
    H_x3_c = P1*fenzi_a/fenmu;
    H_x3_d = P2*fenzi_b;
    H_x3 = H_x3_a+H_x3_b+H_x3_c+H_x3_d;
    %更新状态
    x1 = x1+Delt_T*V0*fenzi_a/fenmu;
    x2 = x2+Delt_T*V0*fenzi_b;
    x3 = x3+Delt_T*w0;
end
f = abs(P1)+abs(P2)+abs(P3);

a2 = f;
    x_opt2=[Re(1),Re(2),Re(3)];
%==========================================================================展开函数myobj_f  OFF
%%
    if(a2<=Ep)
       kk=0;
       x_opt=x_opt2;
       Result_OB=a2;
    else
       kk=1;
       x_opt=x_opt2;
       Result_OB=2;
    end
end
if(kk==1)
    V0 = V;%保持上一时刻的量
    w0 = w;
    z0 = z;
    lamada0 = lamada;
else %--------------------------------------------------------------结束计算，观测结果 PMP
    P1 = x_opt(1);
    P2 = x_opt(2);
    P3 = x_opt(3);
    fenmu = 1-x2*dot_gamma_s(floor(x1));
    fenzi_a = cos(x3-gamma_s(floor(x1)));
    fenzi_b = sin(x3-gamma_s(floor(x1)));
    %控制量更新
    %求解G(x0)
    H_V_a = 2*Cs_dot*(V0*fenzi_a/fenmu-V_tar)*fenzi_a/fenmu;
    H_V_b = 2*Cy_dot*(V0*fenzi_b^2);
    H_V_c = P1*fenzi_a/fenmu;
    H_V_d = P2*fenzi_b;
    H_V = H_V_a+H_V_b+H_V_c+H_V_d;
    H_w = 2*Ctheta_dot*w0+P3;
    H_z = -Cz/(z0+50)-2*lamada0*z0;
    H_lamada = (x1-30)^2/16+(x2-0.5)^2/4-1-z0^2;
    G_x0 = [H_V;H_w;H_z;H_lamada];
    %求解个G(x0+dotx)
    x1_tem = x1+Delt_T*V0*fenzi_a/fenmu;
    x2_tem = x2+Delt_T*V0*fenzi_b;
    x3_tem = x3+Delt_T*w0;
    fenmu_tem = 1-x2_tem*dot_gamma_s(floor(x1_tem));
    fenzi_a_tem = cos(x3_tem-gamma_s(floor(x1_tem)));
    fenzi_b_tem = sin(x3_tem-gamma_s(floor(x1_tem)));
    H_V_a = 2*Cs_dot*(V0*fenzi_a_tem/fenmu_tem-V_tar)*fenzi_a_tem/fenmu_tem;
    H_V_b = 2*Cy_dot*(V0*fenzi_b_tem^2);
    H_V_c = P1*fenzi_a_tem/fenmu_tem;
    H_V_d = P2*fenzi_b_tem;
    H_V_xdot = H_V_a+H_V_b+H_V_c+H_V_d;
    H_w_xdot = 2*Ctheta_dot*w0+P3;
    H_z_xdot = -Cz/(z0+eplim)-2*lamada0*z0;
    H_lamada_dot = (x1_tem-30)^2/16+(x2_tem-0.5)^2/4-1-z0^2;
    G_xdot = [H_V_xdot;H_w_xdot;H_z_xdot;H_lamada_dot];
    G_x_xdot = (G_xdot-G_x0)/0.02;
    %求解G对U的偏导
    G_U_a = 2*Cs_dot*(fenzi_a/fenmu)^2+2*Cy_dot*fenzi_b^2;
    G_U_b = 2*Ctheta_dot;
    G_U_c = -Cz/((z0+eplim)^2)-2*lamada0;
    G_U_d = -2*z0;
    G_U = [G_U_a,0,0,0;0,G_U_b,0,0;0,0,G_U_c,G_U_d;0,0,G_U_d,0];
    %求解u的导数
    dot_u = inv(G_U)*(-G_x_xdot-50*G_x0);
    V0 = V0+dot_u(1)*Delt_T;
    w0 = w0+dot_u(2)*Delt_T;
    z0 = z0+dot_u(3)*Delt_T;
    lamada0 = lamada0+dot_u(4)*Delt_T;
end
    V0 = V0+dot_u(1)*Delt_T
    w0 = w0+dot_u(2)*Delt_T
    z0 = z0+dot_u(3)*Delt_T;
    lamada0 = lamada0+dot_u(4)*Delt_T;

    Result_In=Re(4);
    Flag = kk;
